simulink model "multipath_path_channel"  (R2017b)
settings: Solver=VariableStepAuto  StartTime=0.0  StopTime=10.0  RelTol=1e-3
undefined symbols (not defined in the file or in its folder): doppler
libraries: commchan3 x2, commrandsrc3 x1, commdigbbndpm3 x1
settings Model: Creator=gmuadmin  LastModifiedBy=gmuadmin

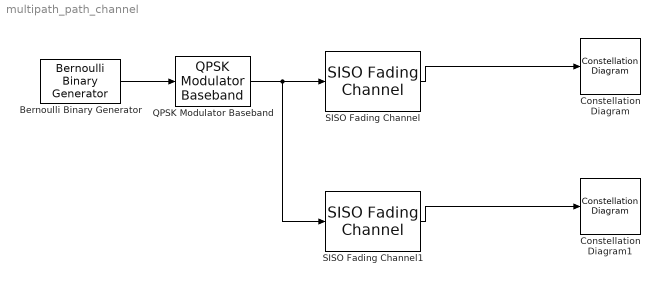
== system multipath_path_channel ==
  Bernoulli Binary Generator : commrandsrc3/Bernoulli Binary Generator  ProbabilityOfZero=0.5  SeedSource=Auto  Seed=0  SampleTime=1/10000000  SamplesPerFrame=2000  OutputDataType=double  SimulateUsing=Interpreted execution
  Constellation Diagram : ConstellationDiagram
  Constellation Diagram1 : ConstellationDiagram
  QPSK Modulator Baseband : commdigbbndpm3/QPSK Modulator Baseband  InType=Integer  Enc=Gray  Ph=pi/4  outDtype=double  outWordLen=16  outUDDataType=sfix(16)  outFracLenMode=Best precision  outFracLen=15  outDataTypeStr=double  outLastDataTypeStr=double
  SISO Fading Channel : commchan3/SISO Fading Channel  PathDelays="1.0e-06 *[0    0.2000    0.4000    0.8000]"  AveragePathGains="[0    -3    -6    -9]"  NormalizePathGains=on  FadingDistribution=Rayleigh  KFactor=3  DirectPathDopplerShift=0  DirectPathInitialPhase=0  MaximumDopplerShift=200  DopplerSpectrum=doppler('Jakes')  RandomStream=mt19937ar with seed  RandomNumGenerator=mt19937ar  Seed=73  PathGainsOutputPort=off  ChannelFilterDelayOutputPort=off  SimulateUsing=Interpreted execution  Visualization=Impulse and frequency responses  PathsForDopplerDisplay=1  SamplesToDisplay=25%
      settings: SourceProductName=Communications System Toolbox
  SISO Fading Channel1 : commchan3/SISO Fading Channel  PathDelays="1.0e-06 *[0    0.2000    0.4000    0.8000]"  AveragePathGains="[0    -3    -6    -9]"  NormalizePathGains=on  FadingDistribution=Rician  KFactor=10  DirectPathDopplerShift=100  DirectPathInitialPhase=0  MaximumDopplerShift=200  DopplerSpectrum=doppler('Jakes')  RandomStream=mt19937ar with seed  RandomNumGenerator=mt19937ar  Seed=73  PathGainsOutputPort=off  ChannelFilterDelayOutputPort=off  SimulateUsing=Interpreted execution  Visualization=Impulse and frequency responses  PathsForDopplerDisplay=1  SamplesToDisplay=25%
      settings: SourceProductName=Communications System Toolbox
  wires:
  Bernoulli Binary Generator/1 -> QPSK Modulator Baseband/1
  QPSK Modulator Baseband/1 -> SISO Fading Channel1/1, SISO Fading Channel/1
  SISO Fading Channel/1 -> Constellation Diagram/1
  SISO Fading Channel1/1 -> Constellation Diagram1/1
